simulink model "prob2"  (R2020b)
settings: Solver=VariableStepAuto  StartTime=0.0  StopTime=100  MaxStep=0.001  RelTol=1e-3
model workspace (MAT data in the model file):
  b = Simulink.Parameter
  b.Value = 50
  b.DataType = 'auto'
  b.Dimensions = [1 1]
  k1 = Simulink.Parameter
  k1.Value = 100
  k1.DataType = 'auto'
  k1.Dimensions = [1 1]
  k2 = Simulink.Parameter
  k2.Value = 200
  k2.DataType = 'auto'
  k2.Dimensions = [1 1]
  m1 = Simulink.Parameter
  m1.Value = 500
  m1.DataType = 'auto'
  m1.Dimensions = [1 1]
  m2 = Simulink.Parameter
  m2.Value = 100
  m2.DataType = 'auto'
  m2.Dimensions = [1 1]
values from neighbouring files (symbols this model uses):
  b = 50    [data2.m]
  k1 = 100    [data2.m]
  k2 = 50    [data2.m]
  m1 = 500    [data2.m]
  m2 = 100    [data2.m]
settings Model: OrderedModelArguments=off  Creator=deves  LastModifiedBy=deves

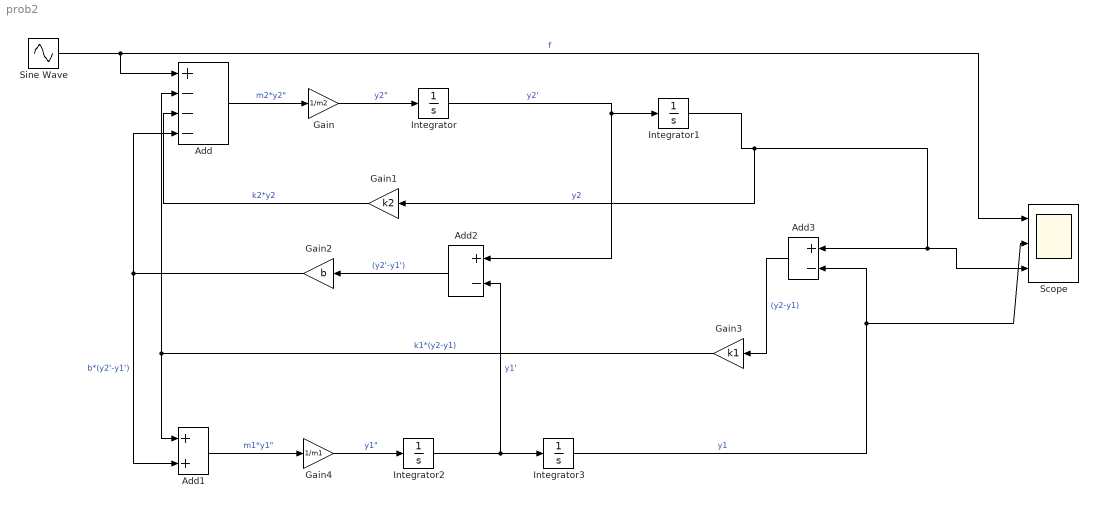
== system prob2 ==
  Add : Sum  Inputs=+---
  Add1 : Sum
  Add2 : Sum  Inputs=+-
  Add3 : Sum  Inputs=+-
  Gain : Gain  Gain=1/m2
  Gain1 : Gain  Gain=k2
  Gain2 : Gain  Gain=b
  Gain3 : Gain  Gain=k1
  Gain4 : Gain  Gain=1/m1
  Integrator{,1..3} (4 alike) : Integrator
  Scope : Scope  NumInputPorts=3
  Sine Wave : Sin  Amplitude=5  SampleTime=0
  wires:
  Add/1 -> Gain/1  "m2*y2\""
  Add1/1 -> Gain4/1  "m1*y1\""
  Gain4/1 -> Integrator2/1  "y1\""
  Integrator2/1 -> Add2/2, Integrator3/1  "y1'"
  Gain/1 -> Integrator/1  "y2\""
  Integrator/1 -> Add2/1, Integrator1/1  "y2'"
  Integrator3/1 -> Add3/2, Scope/2  "y1"
  Integrator1/1 -> Gain1/1, Scope/3, Add3/1  "y2"
  Add3/1 -> Gain3/1  "(y2-y1)"
  Add2/1 -> Gain2/1  "(y2'-y1')"
  Gain2/1 -> Add/4, Add1/2  "b*(y2'-y1')"
  Gain3/1 -> Add1/1, Add/2  "k1*(y2-y1)"
  Gain1/1 -> Add/3  "k2*y2"
  Sine Wave/1 -> Add/1, Scope/1  "f"
